simulink model "OLD_UAV_Dynamics_Autopilot_Communication"  (R2023b)
settings: Solver=ode4  StartTime=0.0  StopTime=inf  FixedStep=1/500  RelTol=1e-3
values from neighbouring files (symbols this model uses):
  dragCoeffMov = 0.01    [InitHexacopterPlantVars.m]
  m_to_mm = 1000    [InitHexacopterPlantVars.m]
  ms_to_cms = 100    [InitHexacopterPlantVars.m]
  ref_height = 23    [InitHexacopterPlantVars.m]
  ref_lat = 36.364905    [InitHexacopterPlantVars.m]
  ref_lon = 127.344377    [InitHexacopterPlantVars.m]
  rotorDir = [1 -1 1 -1 -1 1]    [InitHexacopterPlantVars.m]
  rotorPositions = zeros(3,6)    [InitHexacopterPlantVars.m]
  rotorThrustMax = 4    [InitHexacopterPlantVars.m]
  rotorTimeConst = 0.050    (= 0.05)    [InitHexacopterPlantVars.m]
  rotorTorqueMax = 0.05    [InitHexacopterPlantVars.m]
  SampleTime = 1/100    (= 0.01)    [InitHexacopterPlantVars.m]
  Ts_sensor = 1/100    (= 0.01)    [InitHexacopterPlantVars.m]
  uT_to_gauss = 0.01    [InitHexacopterPlantVars.m]
  windVel = [0 0 0]'    [InitHexacopterPlantVars.m]
  x0 = [0 0 0 0 0 0 0 0 0 0 0 0]    [InitHexacopterPlantVars.m]
undefined symbols (not defined in the file or in its folder): contact, control, ddx, ddy, ddz, dx, dy, dz, earthRadius, fractalcoef, g, Mass, p, Payload, pitch, q, r, r2d, Receive, roll, Send, X, Y, yaw, Z
libraries: uavmavlinklib x7, aerolibfltsims x3, px4MAVLinkBridgelib x2, aerolibanimutils x2, simulink x2, aerolibatmos2 x1, sensorgpslib x1, robotcorelib x1, mspsensorlib x1, aerolibasang x1, shared6dof x1
(part 2 of 2)

== matlab function OLD_UAV_Dynamics_Autopilot_Communication/Subsystem/Subsystem/Quadcopter Model1/Force and Moment Calculation/Rotor Model/MATLAB Function ==
  data: thrustEachRotor input; tauEachRotor input; rotorPositions input; netF output; netM output; rotorDir input
function [netF, netM] = getForceMoment(thrustEachRotor, tauEachRotor, rotorPositions, rotorDir)
%#codegen
Fx = 0;
Fy = 0;
Fz = -sum(thrustEachRotor);

netF = [Fx; Fy; Fz];

netM = [0; 0; 0]; %initialize
    for i = 1:6
        rotPos = rotorPositions(:, i);
        Fi = [0, 0, -thrustEachRotor(i)]';
        netM = netM +  cross(rotPos, Fi);%contribution from thrusts of each propeller
        netM(3) = netM(3) - rotorDir(i)*tauEachRotor(i); %contribution from counter torque acting on propeller
    end

end
